simulink model "Number_4"  (R2023b)
settings: Solver=VariableStepAuto  StartTime=0.0  StopTime=20  RelTol=1e-3
values from neighbouring files (symbols this model uses):
  G_den4 = [1 1]    [Number_3_4.m]
  G_num4 = [1]    [Number_3_4.m]
settings Model: Creator=Corinne  LastModifiedBy=Corinne

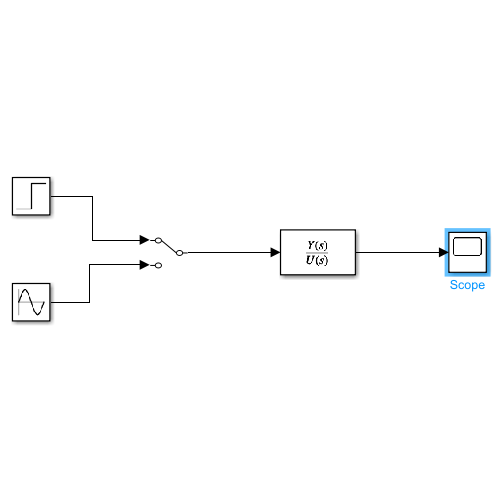
[thumbnail: Simulink's stored preview of the top-level diagram]
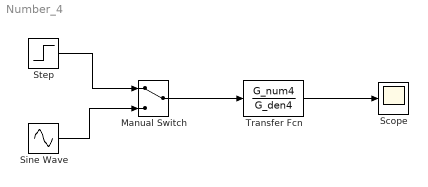
== system Number_4 ==
  Manual Switch : ManualSwitch
  Scope : Scope
  Sine Wave : Sin  SampleTime=0
  Step : Step  Time=0  SampleTime=0
  Transfer Fcn : TransferFcn  Numerator=G_num4  Denominator=G_den4
  wires:
  Step/1 -> Manual Switch/1
  Sine Wave/1 -> Manual Switch/2
  Manual Switch/1 -> Transfer Fcn/1
  Transfer Fcn/1 -> Scope/1
